simulink model "components"  (R2014a)
settings: Solver=ode45  StartTime=0.0  StopTime=10.0  RelTol=1e-3
libraries: simulink x3, commnoisgen2 x2, dspspect3 x2, dspxfrm3 x1, simrfV2elements x1, rfmathmodels1 x1, rfphysmodels1 x1, commsource2 x1
settings Model: Creator=zain  LastModifiedBy=zain

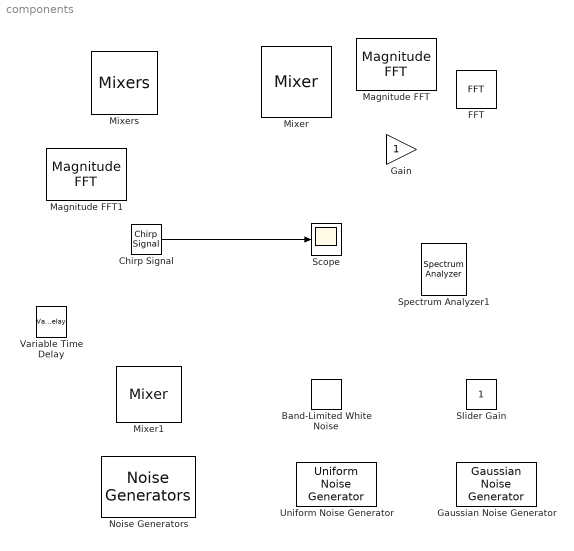
== system components ==
  Band-Limited White Noise : simulink/Sources/Band-Limited White Noise  Cov=[0.1]  Ts=0.1  seed=[23341]
  Chirp Signal : simulink/Sources/Chirp Signal  f1=4500000000  T=0.25  f2=6000000000
  FFT : dspxfrm3/FFT  CompMethod=Table lookup  TableOpt=NEW  TableOptActive=Speed  BitRevOrder=off  InheritFFTLength=on  FFTLength=64  WrapInput=on  RowConvenienceOn=on  FFTImplementation=Auto  SkipNorm=off  firstCoeffDataTypeStr=Inherit: Same word length as input  firstCoeffLastDataTypeStr=Inherit: Same word length as input  outputMin=[]  outputMax=[]  roundingMode=Floor  overflowMode=off
  Gain : Gain
  Gaussian Noise Generator : commnoisgen2/Gaussian Noise Generator  m=0  d=1  s=41  Ts=1  frameBased=off  sampPerFrame=1  orient=off  outDataType=double
  Magnitude FFT : dspspect3/Magnitude FFT  mag_or_magsq=Magnitude squared  FFTImplementation=Auto  fftLenInherit=off  fftsize=256  WrapInput=on
  Magnitude FFT1 : dspspect3/Magnitude FFT  mag_or_magsq=Magnitude squared  FFTImplementation=Auto  fftLenInherit=off  fftsize=256  WrapInput=on
  Mixer : simrfV2elements/Mixer  classname=mixer  Source_linear_gain=Available power gain  linear_gain=0 dB  Zin=50  Zout=50  ZLO=inf  Source_Poly=Even and odd order  Poly_Coeffs=[0 1]  IPType=Output  IP2=Inf dBm  IP3=Inf dBm  P1dB=Inf dBm  Psat=Inf dBm  Gcomp=Inf dBm  NF=0  InternalGrounding=on
  Mixer1 : rfmathmodels1/Mixer  gain=0  PhNs=-120  Fo=100  seed=2137  loss=0
  Mixers : rfphysmodels1/Mixers  SystemSampleTime=-1
  Noise Generators : commsource2/Noise Generators
  Scope : Scope
  Slider Gain : simulink/Math Operations/Slider Gain  low=0  gain=1  high=2
  Spectrum Analyzer1 : SpectrumAnalyzer
  Uniform Noise Generator : commnoisgen2/Uniform Noise Generator  low=0  up=1  seed=31  Ts=1  frameBased=off  sampPerFrame=1  orient=off  outDataType=double
  Variable Time Delay : VariableTransportDelay  MaximumDelay=10
  wires:
  Chirp Signal/1 -> Scope/1
